simulink model "integrator_single_double_compare"  (R2021b)
settings: Solver=VariableStepAuto  StartTime=0.0  StopTime=1  RelTol=1e-3
undefined symbols (not defined in the file or in its folder): DiscIntNeverNeededParam
libraries: slpidlib x7
settings Model: Creator=ts  LastModifiedBy=ts

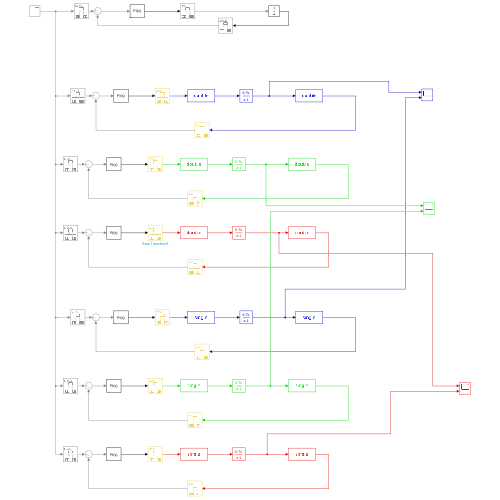
[thumbnail: Simulink's stored preview of the top-level diagram]
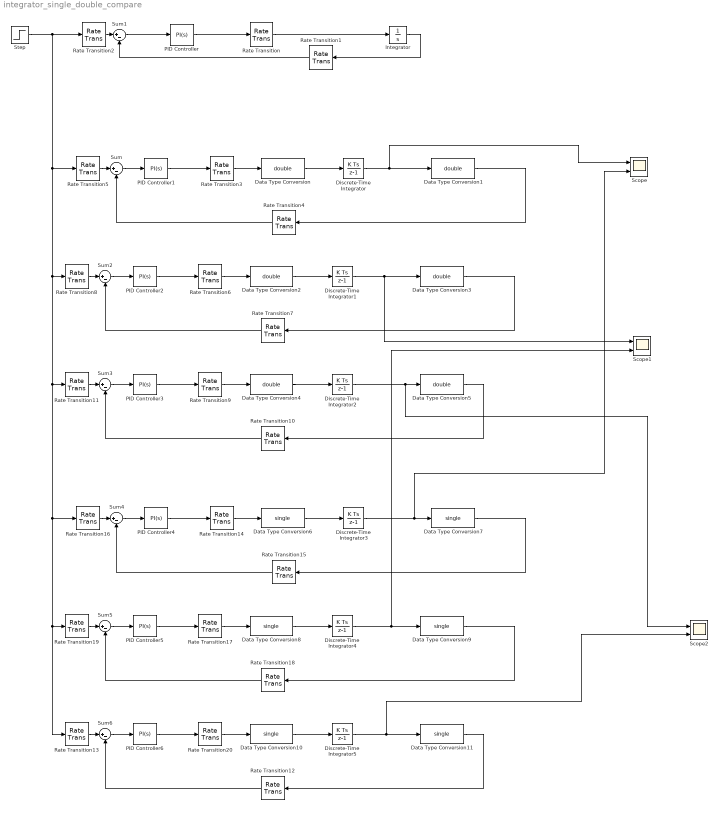
== system integrator_single_double_compare ==
  Data Type Conversion{,1..5} (6 alike) : DataTypeConversion  OutDataTypeStr=double
  Data Type Conversion{6..11} (6 alike) : DataTypeConversion  OutDataTypeStr=single
  Discrete-Time Integrator{,1..5} (6 alike) : DiscreteIntegrator  SampleTime=-1  ICPrevOutput=DiscIntNeverNeededParam  ICPrevScaledInput=DiscIntNeverNeededParam
  Integrator : Integrator
  PID Controller{,1..6} (7 alike) : slpidlib/PID Controller  Controller=PI  Form=Parallel  TimeDomain=Continuous-time  UseExternalTs=off  SampleTime=-1  IntegratorMethod=Forward Euler  FilterMethod=Forward Euler  ControllerParametersSource=internal  P=1  I=1  D=0  UseFilter=on  N=100  TunerSelectOption=Transfer Function Based (PID Tuner App)  InitialConditionSource=internal  InitialConditionForIntegrator=0  InitialConditionForFilter=0  DifferentiatorICPrevScaledInput=0  ExternalReset=none  TrackingMode=off  Kt=1  LimitOutput=off  SatLimitsSource=internal  UpperSaturationLimit=inf  LowerSaturationLimit=-inf  LinearizeAsGain=on  AntiWindupMode=none  Kb=1  POutMin=[]  POutMax=[]  IOutMin=[]  IOutMax=[]  DOutMin=[]  DOutMax=[]  NOutMin=[]  NOutMax=[]  SumOutMin=[]  SumOutMax=[]  SaturationOutMin=[]  SaturationOutMax=[]  PParamMin=[]  PParamMax=[]  IParamMin=[]  IParamMax=[]  DParamMin=[]  DParamMax=[]  NParamMin=[]  NParamMax=[]  KbParamMin=[]  KbParamMax=[]  KtParamMin=[]  KtParamMax=[]  KbOutMin=[]  KbOutMax=[]  KtOutMin=[]  KtOutMax=[]  IntegratorOutMin=[]  IntegratorOutMax=[]  FilterOutMin=[]  FilterOutMax=[]  SumI1OutMin=[]  SumI1OutMax=[]  SumI2OutMin=[]  SumI2OutMax=[]  SumI3OutMin=[]  SumI3OutMax=[]  SumI4OutMin=[]  SumI4OutMax=[]  SumDOutMin=[]  SumDOutMax=[]  DifferentiatorOutMin=[]  DifferentiatorOutMax=[]  FilterDiffOutCoefMin=[]  FilterDiffOutCoefMax=[]  ReciprocalOutMin=[]  ReciprocalOutMax=[]  SumDenOutMin=[]  SumDenOutMax=[]  SumNumOutMin=[]  SumNumOutMax=[]  DivideOutMin=[]  DivideOutMax=[]  UdiffTsProdOutMin=[]  UdiffTsProdOutMax=[]  NTsProdOutMin=[]  NTsProdOutMax=[]  UintegralTsProdOutMin=[]  UintegralTsProdOutMax=[]  UngainTsProdOutMin=[]  UngainTsProdOutMax=[]  IntegratorContinuousStateAttributes=''  IntegratorStateMustResolveToSignalObject=off  IntegratorRTWStateStorageClass=Auto  FilterContinuousStateAttributes=''  FilterStateMustResolveToSignalObject=off  FilterRTWStateStorageClass=Auto  ParallelPVariant=InternalParameters  IdealPVariant=Disabled  IVariant=InternalParameters  DVariant=Disabled  IntegratorVariant=Continuous  SatVariant=Disabled  AWVariant=Passthrough  PCopyVariant=Disabled  TRVariant=Disabled  FdbkBlocksVariant=Forward  IdealPFdbkVariant=Disabled  SatFdbkVariant=Disabled  DerivativeFilterVariant=Disabled  NVariant=Disabled  NCopyVariant=Disabled_SignalSpec  FilterICVariant=Disabled  IntegratorICVariant=InternalICs  ExternalResetVariant=Disabled  TRSumVariant=Passthrough  SumFdbkVariant=Disabled  SumVariant=Sum_PI  TsampFilterVariant=InternalTs  TsampNgainVariant=Passthrough  TsampIntegralVariant=Passthrough  ExternalSaturationOutDataTypeStr=Inherit: Same as second input
  Rate Transition{,1..2,4..5,7..8,10..13,15..16,18..19} (15 alike) : RateTransition
  Rate Transition14 : RateTransition  OutPortSampleTime=1/1e6
  Rate Transition17 : RateTransition  OutPortSampleTime=1/10e6
  Rate Transition20 : RateTransition  OutPortSampleTime=1/100e6
  Rate Transition3 : RateTransition  OutPortSampleTime=1/1e6
  Rate Transition6 : RateTransition  OutPortSampleTime=1/10e6
  Rate Transition9 : RateTransition  OutPortSampleTime=1/100e6
  Scope : Scope  NumInputPorts=2
  Scope1 : Scope  NumInputPorts=2
  Scope2 : Scope  NumInputPorts=2
  Step : Step  Time=0.001  SampleTime=0
  Sum{,1..6} (7 alike) : Sum  Inputs=|+-
  wires:
  Sum/1 -> PID Controller1/1
  Sum1/1 -> PID Controller/1
  PID Controller/1 -> Rate Transition/1
  Rate Transition/1 -> Integrator/1
  Integrator/1 -> Rate Transition1/1
  Rate Transition1/1 -> Sum1/2
  Rate Transition2/1 -> Sum1/1
  PID Controller1/1 -> Rate Transition3/1
  Discrete-Time Integrator/1 -> Scope/1, Data Type Conversion1/1
  Rate Transition3/1 -> Data Type Conversion/1
  Rate Transition4/1 -> Sum/2
  Rate Transition5/1 -> Sum/1
  Data Type Conversion/1 -> Discrete-Time Integrator/1
  Data Type Conversion1/1 -> Rate Transition4/1
  Discrete-Time Integrator1/1 -> Scope1/1, Data Type Conversion3/1
  Rate Transition8/1 -> Sum2/1
  Data Type Conversion2/1 -> Discrete-Time Integrator1/1
  Rate Transition7/1 -> Sum2/2
  Rate Transition6/1 -> Data Type Conversion2/1
  Data Type Conversion3/1 -> Rate Transition7/1
  PID Controller2/1 -> Rate Transition6/1
  Sum2/1 -> PID Controller2/1
  Discrete-Time Integrator2/1 -> Scope2/1, Data Type Conversion5/1
  Rate Transition11/1 -> Sum3/1
  Data Type Conversion4/1 -> Discrete-Time Integrator2/1
  Rate Transition10/1 -> Sum3/2
  Rate Transition9/1 -> Data Type Conversion4/1
  Data Type Conversion5/1 -> Rate Transition10/1
  PID Controller3/1 -> Rate Transition9/1
  Sum3/1 -> PID Controller3/1
  PID Controller6/1 -> Rate Transition20/1
  Data Type Conversion11/1 -> Rate Transition12/1
  Discrete-Time Integrator5/1 -> Scope2/2, Data Type Conversion11/1
  PID Controller5/1 -> Rate Transition17/1
  Rate Transition17/1 -> Data Type Conversion8/1
  Rate Transition18/1 -> Sum5/2
  Rate Transition20/1 -> Data Type Conversion10/1
  Rate Transition19/1 -> Sum5/1
  Rate Transition14/1 -> Data Type Conversion6/1
  Rate Transition12/1 -> Sum6/2
  Step/1 -> Rate Transition2/1, Rate Transition13/1, Rate Transition19/1, Rate Transition16/1, Rate Transition11/1, Rate Transition8/1, Rate Transition5/1
  Data Type Conversion8/1 -> Discrete-Time Integrator4/1
  Sum6/1 -> PID Controller6/1
  Rate Transition15/1 -> Sum4/2
  Data Type Conversion6/1 -> Discrete-Time Integrator3/1
  Rate Transition16/1 -> Sum4/1
  Data Type Conversion7/1 -> Rate Transition15/1
  Discrete-Time Integrator4/1 -> Scope1/2, Data Type Conversion9/1
  Rate Transition13/1 -> Sum6/1
  Data Type Conversion9/1 -> Rate Transition18/1
  Sum5/1 -> PID Controller5/1
  Data Type Conversion10/1 -> Discrete-Time Integrator5/1
  Discrete-Time Integrator3/1 -> Scope/2, Data Type Conversion7/1
  PID Controller4/1 -> Rate Transition14/1
  Sum4/1 -> PID Controller4/1
